simulink model "BlockDiagram"  (R2016b)
settings: Solver=VariableStepAuto  StartTime=0.0  StopTime=10.0  RelTol=1e-3
values from neighbouring files (symbols this model uses):
  a = 5.78*10^-1    (= 0.578)    [scriptBE125.m]
  b = 3.91*10^-4    (= 0.000391)    [scriptBE125.m]
  N = 200    [Beng125ModelandParam.m]    (also in Beng125ModelandParam_version2.m; Beng125model.m; scriptBE125.m)
undefined symbols (not defined in the file or in its folder): y
settings Model: Creator=myemle  LastModifiedBy=myemle

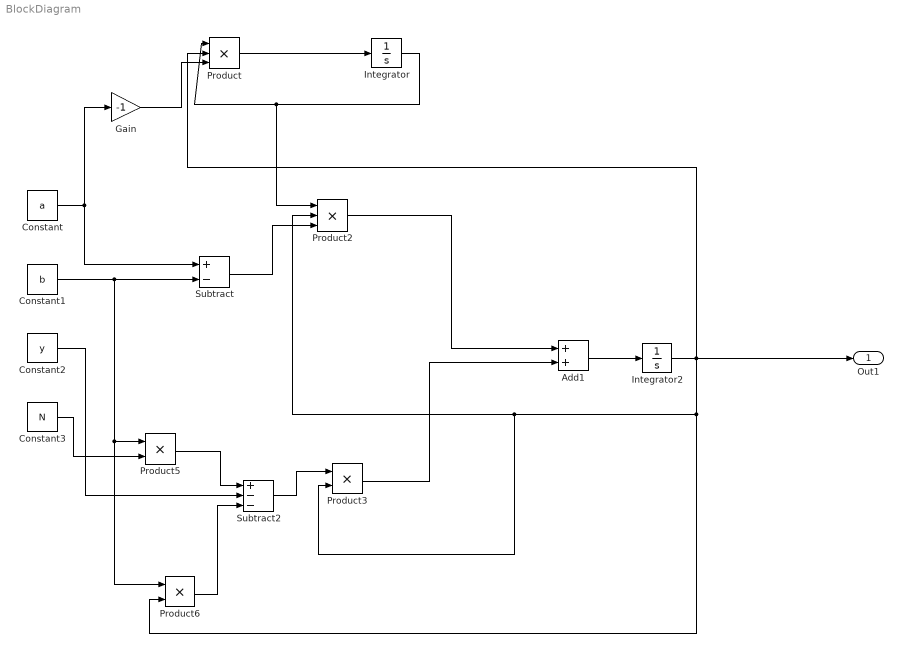
== system BlockDiagram ==
  Add1 : Sum
  Constant : Constant  Value=a
  Constant1 : Constant  Value=b
  Constant2 : Constant  Value=y
  Constant3 : Constant  Value=N
  Gain : Gain  Gain=-1
  Integrator : Integrator  InitialCondition=198
  Integrator2 : Integrator  InitialCondition=2
  Product : Product  Inputs=3
  Product2 : Product  Inputs=3
  Product3 : Product
  Product5 : Product
  Product6 : Product
  Subtract : Sum  Inputs=+-
  Subtract2 : Sum  Inputs=+--
  Out1 : Outport
  wires:
  Integrator/1 -> Product2/1, Product/1
  Product3/1 -> Add1/2
  Product2/1 -> Add1/1
  Add1/1 -> Integrator2/1
  Integrator2/1 -> Product6/2, Product2/2, Product3/2, Out1/1, Product/2
  Constant/1 -> Subtract/1, Gain/1
  Gain/1 -> Product/3
  Subtract2/1 -> Product3/1
  Product5/1 -> Subtract2/1
  Constant3/1 -> Product5/2
  Constant2/1 -> Subtract2/2
  Constant1/1 -> Product6/1, Product5/1, Subtract/2
  Product6/1 -> Subtract2/3
  Product/1 -> Integrator/1
  Subtract/1 -> Product2/3
